simulink model "BusTest"  (R2022b)
settings: Solver=VariableStepAuto  StartTime=0.0  StopTime=10.0  RelTol=1e-3
undefined symbols (not defined in the file): AB_SAMPLE, ABC_SAMPLE, AC_SAMPLE, C_Fault_IaConfirmCnt_u16, C_Fault_IaInstantFaultCoeff_f32, C_Fault_IaInstantFaultDiagEn_u8, C_Fault_IaInstantFaultLevel_u8, ParamCfg_LaValueDefault_u16, ParamCfg_SampleMode_u16
libraries: simulink x4
settings Model: Creator=ZYH  LastModifiedBy=ZYH

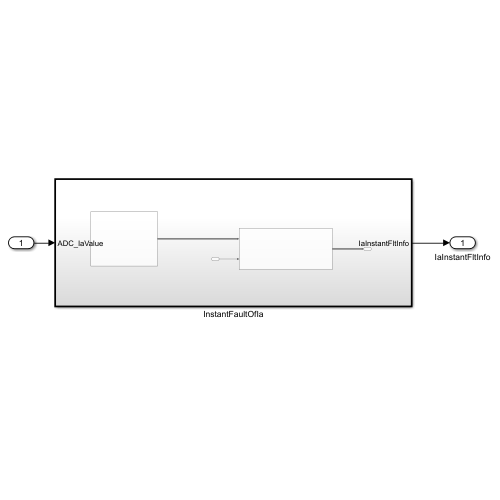
[thumbnail: Simulink's stored preview of the top-level diagram]
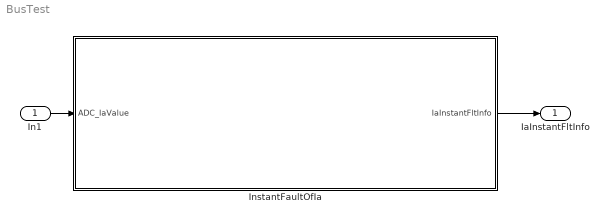
== system BusTest ==
  In1 : Inport
  InstantFaultOfIa : Subsystem  TreatAsAtomicUnit=on
      settings: RTWSystemCode=Nonreusable function
  IaInstantFltInfo : Outport
  wires:
  In1/1 -> InstantFaultOfIa/1(ADC_IaValue)
  InstantFaultOfIa/1(IaInstantFltInfo) -> IaInstantFltInfo/1

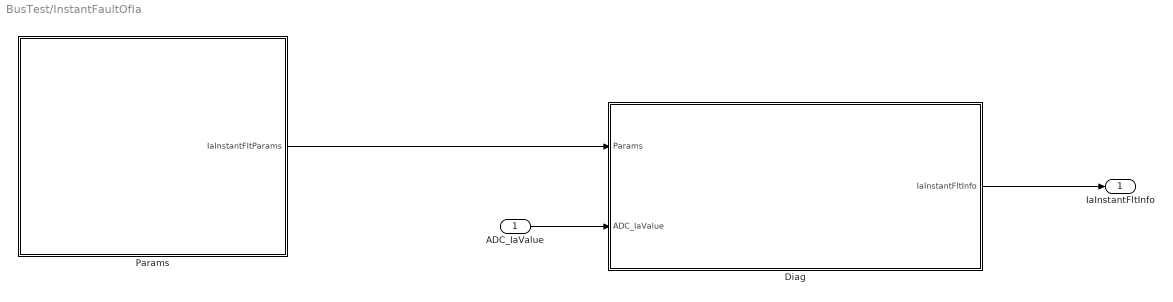
== system BusTest/InstantFaultOfIa ==
  ADC_IaValue : Inport
  Diag : Subsystem
  Params : Subsystem
  IaInstantFltInfo : Outport
  wires:
  Params/1(IaInstantFltParams) -> Diag/1(Params)
  ADC_IaValue/1 -> Diag/2(ADC_IaValue)
  Diag/1(IaInstantFltInfo) -> IaInstantFltInfo/1

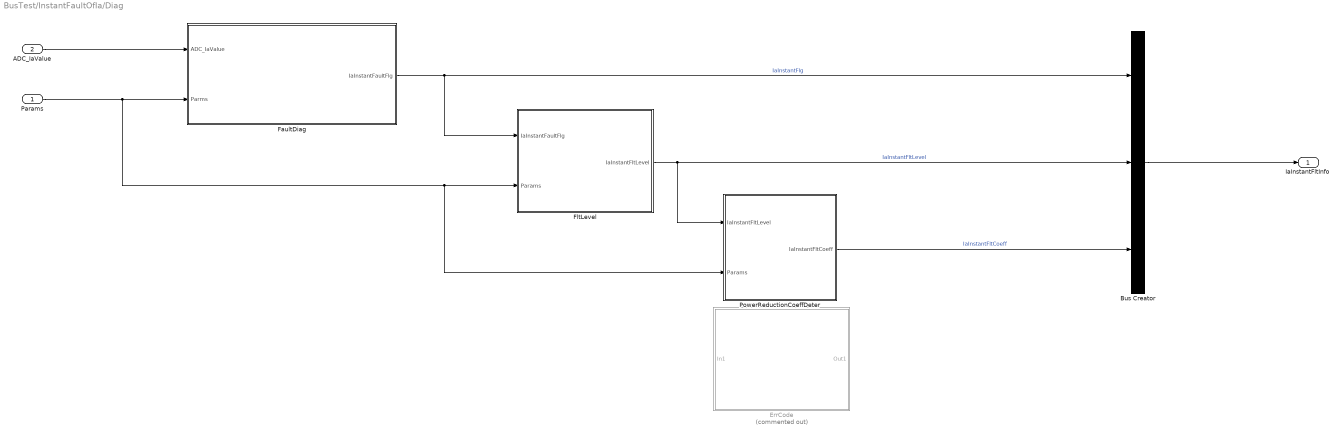
== system BusTest/InstantFaultOfIa/Diag ==
  Params : Inport
  ADC_IaValue : Inport  Port=2
  Bus Creator : BusCreator  Inputs=3  OutDataTypeStr=Bus: FaultBus
      settings: InheritFromInputs=off
  ErrCode : Subsystem  Commented=on
  FaultDiag : Subsystem
  FltLevel : Subsystem
  PowerReductionCoeffDeter : Subsystem
  IaInstantFltInfo : Outport
  wires:
  Params/1 -> PowerReductionCoeffDeter/2(Params), FltLevel/2(Params), FaultDiag/2(Parms)
  ADC_IaValue/1 -> FaultDiag/1(ADC_IaValue)
  FaultDiag/1(IaInstantFaultFlg) -> FltLevel/1(IaInstantFaultFlg), Bus Creator/1  "IaInstantFlg"
  PowerReductionCoeffDeter/1(IaInstantFltCoeff) -> Bus Creator/3  "IaInstantFltCoeff"
  FltLevel/1(IaInstantFltLevel) -> PowerReductionCoeffDeter/1(IaInstantFltLevel), Bus Creator/2  "IaInstantFltLevel"
  Bus Creator/1 -> IaInstantFltInfo/1

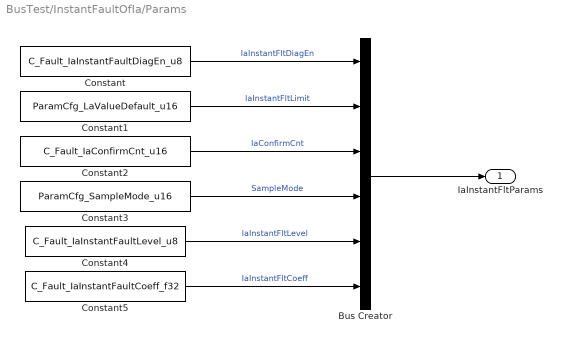
== system BusTest/InstantFaultOfIa/Params ==
  Bus Creator : BusCreator  Inputs=6
  Constant : Constant  Value=C_Fault_IaInstantFaultDiagEn_u8
  Constant1 : Constant  Value=ParamCfg_LaValueDefault_u16
  Constant2 : Constant  Value=C_Fault_IaConfirmCnt_u16  OutDataTypeStr=uint16
  Constant3 : Constant  Value=ParamCfg_SampleMode_u16
  Constant4 : Constant  Value=C_Fault_IaInstantFaultLevel_u8
  Constant5 : Constant  Value=C_Fault_IaInstantFaultCoeff_f32
  IaInstantFltParams : Outport
  wires:
  Constant1/1 -> Bus Creator/2  "IaInstantFltLimit"
  Constant/1 -> Bus Creator/1  "IaInstantFltDiagEn"
  Constant2/1 -> Bus Creator/3  "IaConfirmCnt"
  Bus Creator/1 -> IaInstantFltParams/1
  Constant3/1 -> Bus Creator/4  "SampleMode"
  Constant4/1 -> Bus Creator/5  "IaInstantFltLevel"
  Constant5/1 -> Bus Creator/6  "IaInstantFltCoeff"

== system BusTest/InstantFaultOfIa/Diag/ErrCode ==
  In1 : Inport
  Out1 : Outport
  wires:
  In1/1 -> Out1/1

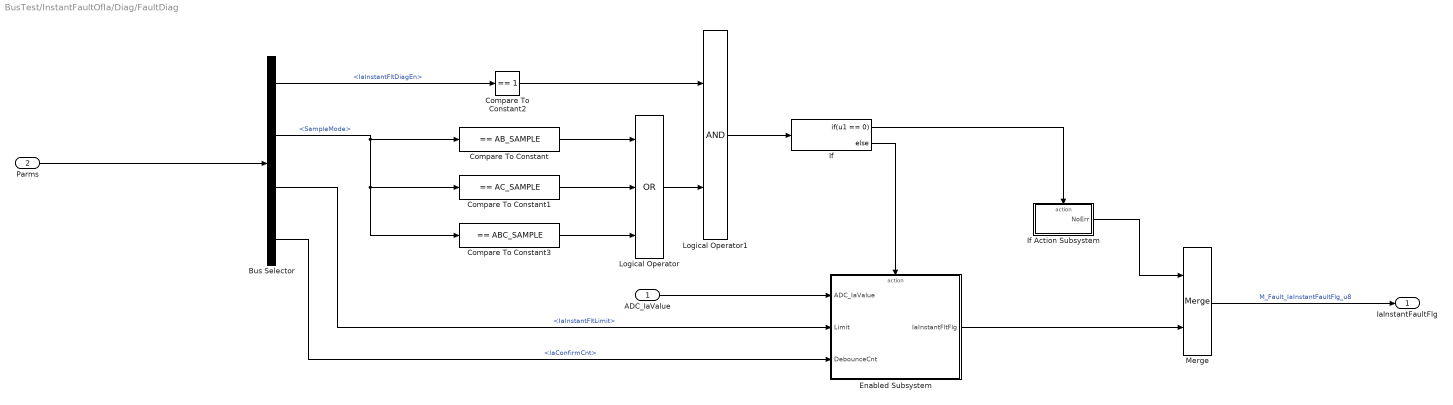
== system BusTest/InstantFaultOfIa/Diag/FaultDiag ==
  ADC_IaValue : Inport
  Parms : Inport  Port=2
  Bus Selector : BusSelector  OutputSignals=IaInstantFltDiagEn,SampleMode,IaInstantFltLimit,IaConfirmCnt
  Compare To Constant : simulink/Logic and Bit Operations/Compare To Constant  relop===  const=AB_SAMPLE  OutDataTypeStr=boolean
  Compare To Constant1 : simulink/Logic and Bit Operations/Compare To Constant  relop===  const=AC_SAMPLE  OutDataTypeStr=boolean
  Compare To Constant2 : simulink/Logic and Bit Operations/Compare To Constant  relop===  const=1  OutDataTypeStr=boolean
  Compare To Constant3 : simulink/Logic and Bit Operations/Compare To Constant  relop===  const=ABC_SAMPLE  OutDataTypeStr=boolean
  Enabled Subsystem : Subsystem  TreatAsAtomicUnit=on
  If : If  IfExpression=u1 == 0
  If Action Subsystem : Subsystem  TreatAsAtomicUnit=on
  Logical Operator : Logic  Operator=OR  Inputs=3  AllPortsSameDT=off  OutDataTypeStr=boolean
  Logical Operator1 : Logic  AllPortsSameDT=off  OutDataTypeStr=boolean
  Merge : Merge
  IaInstantFaultFlg : Outport
  wires:
  ADC_IaValue/1 -> Enabled Subsystem/1(ADC_IaValue)
  Bus Selector/4 -> Enabled Subsystem/3(DebounceCnt)  "<IaConfirmCnt>"
  Compare To Constant2/1 -> Logical Operator1/1
  Bus Selector/2 -> Compare To Constant3/1, Compare To Constant1/1, Compare To Constant/1  "<SampleMode>"
  Bus Selector/1 -> Compare To Constant2/1  "<IaInstantFltDiagEn>"
  Logical Operator/1 -> Logical Operator1/2
  Compare To Constant/1 -> Logical Operator/1
  Logical Operator1/1 -> If/1
  Compare To Constant3/1 -> Logical Operator/3
  Bus Selector/3 -> Enabled Subsystem/2(Limit)  "<IaInstantFltLimit>"
  Enabled Subsystem/1(IaInstantFltFlg) -> Merge/2
  If/2 -> Enabled Subsystem/Action
  Compare To Constant1/1 -> Logical Operator/2
  If Action Subsystem/1(NoErr) -> Merge/1
  If/1 -> If Action Subsystem/Action
  Parms/1 -> Bus Selector/1
  Merge/1 -> IaInstantFaultFlg/1  "M_Fault_IaInstantFaultFlg_u8"

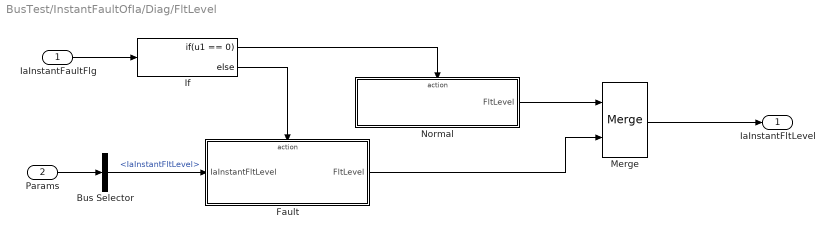
== system BusTest/InstantFaultOfIa/Diag/FltLevel ==
  IaInstantFaultFlg : Inport
  Params : Inport  Port=2
  Bus Selector : BusSelector  OutputSignals=IaInstantFltLevel
  Fault : Subsystem  TreatAsAtomicUnit=on
  If : If  IfExpression=u1 == 0
  Merge : Merge
  Normal : Subsystem  TreatAsAtomicUnit=on
  IaInstantFltLevel : Outport
  wires:
  IaInstantFaultFlg/1 -> If/1
  If/1 -> Normal/Action
  If/2 -> Fault/Action
  Params/1 -> Bus Selector/1
  Bus Selector/1 -> Fault/1(IaInstantFltLevel)  "<IaInstantFltLevel>"
  Normal/1(FltLevel) -> Merge/1
  Fault/1(FltLevel) -> Merge/2
  Merge/1 -> IaInstantFltLevel/1

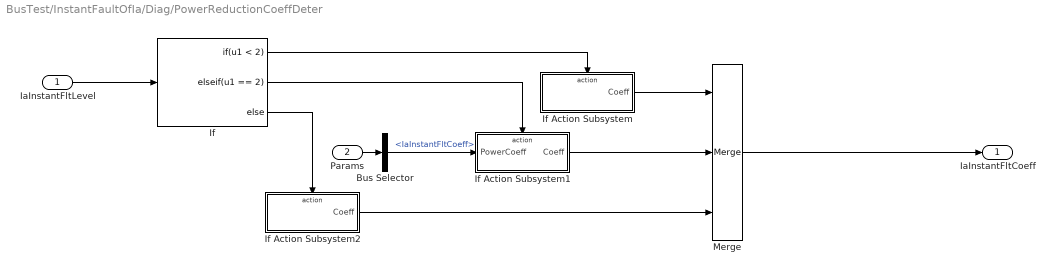
== system BusTest/InstantFaultOfIa/Diag/PowerReductionCoeffDeter ==
  IaInstantFltLevel : Inport
  Params : Inport  Port=2
  Bus Selector : BusSelector  OutputSignals=IaInstantFltCoeff
  If : If  IfExpression=u1 < 2  ElseIfExpressions=u1 == 2
  If Action Subsystem : Subsystem  TreatAsAtomicUnit=on
  If Action Subsystem1 : Subsystem  TreatAsAtomicUnit=on
  If Action Subsystem2 : Subsystem  TreatAsAtomicUnit=on
  Merge : Merge  Inputs=3
  IaInstantFltCoeff : Outport
  wires:
  IaInstantFltLevel/1 -> If/1
  If/1 -> If Action Subsystem/Action
  If/2 -> If Action Subsystem1/Action
  If/3 -> If Action Subsystem2/Action
  If Action Subsystem/1(Coeff) -> Merge/1
  If Action Subsystem1/1(Coeff) -> Merge/2
  If Action Subsystem2/1(Coeff) -> Merge/3
  Merge/1 -> IaInstantFltCoeff/1
  Bus Selector/1 -> If Action Subsystem1/1(PowerCoeff)  "<IaInstantFltCoeff>"
  Params/1 -> Bus Selector/1

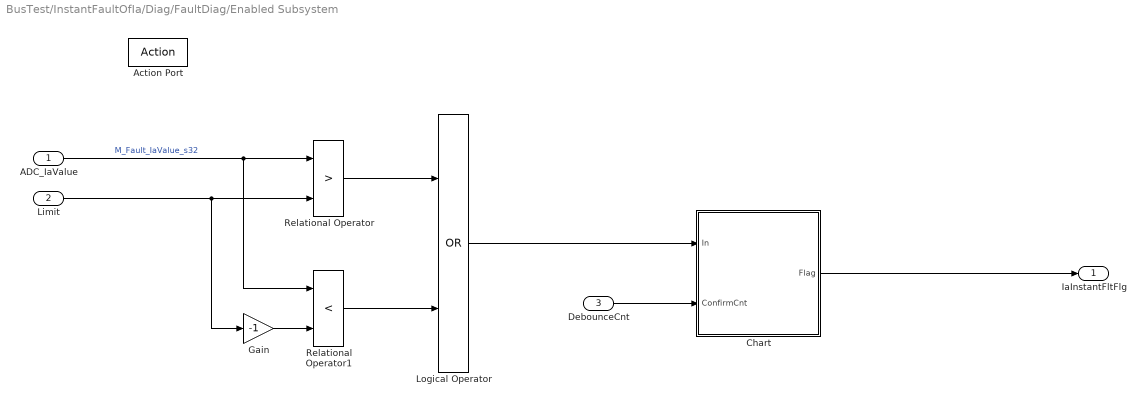
== system BusTest/InstantFaultOfIa/Diag/FaultDiag/Enabled Subsystem ==
  ADC_IaValue : Inport
  Limit : Inport  Port=2
  DebounceCnt : Inport  Port=3
  Action Port : ActionPort
  Chart : Stateflow chart  TreatAsAtomicUnit=on
      settings: RTWSystemCode=Inline
  Gain : Gain  Gain=-1  ParamDataTypeStr=single  OutDataTypeStr=single
  Logical Operator : Logic  Operator=OR  AllPortsSameDT=off  OutDataTypeStr=boolean
  Relational Operator : RelationalOperator  Operator=>  OutDataTypeStr=boolean  RndMeth=Simplest  InputSameDT=off
  Relational Operator1 : RelationalOperator  Operator=<  OutDataTypeStr=boolean  RndMeth=Simplest  InputSameDT=off
  IaInstantFltFlg : Outport
  wires:
  Logical Operator/1 -> Chart/1(In)
  Relational Operator/1 -> Logical Operator/1
  Gain/1 -> Relational Operator1/2
  ADC_IaValue/1 -> Relational Operator1/1, Relational Operator/1  "M_Fault_IaValue_s32"
  Relational Operator1/1 -> Logical Operator/2
  Limit/1 -> Gain/1, Relational Operator/2
  DebounceCnt/1 -> Chart/2(ConfirmCnt)
  Chart/1(Flag) -> IaInstantFltFlg/1

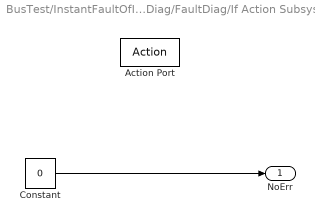
== system BusTest/InstantFaultOfIa/Diag/FaultDiag/If Action Subsystem ==
  Action Port : ActionPort
  Constant : Constant  Value=0  OutDataTypeStr=uint8
  NoErr : Outport
  wires:
  Constant/1 -> NoErr/1

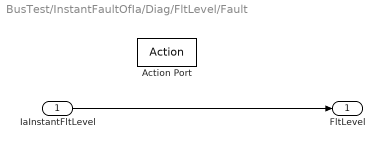
== system BusTest/InstantFaultOfIa/Diag/FltLevel/Fault ==
  IaInstantFltLevel : Inport
  Action Port : ActionPort
  FltLevel : Outport
  wires:
  IaInstantFltLevel/1 -> FltLevel/1

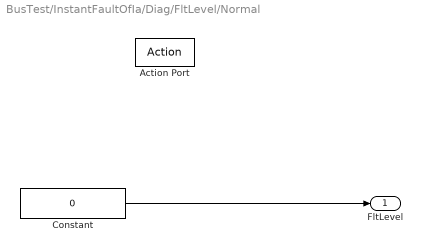
== system BusTest/InstantFaultOfIa/Diag/FltLevel/Normal ==
  Action Port : ActionPort
  Constant : Constant  Value=0  OutDataTypeStr=uint8
  FltLevel : Outport
  wires:
  Constant/1 -> FltLevel/1

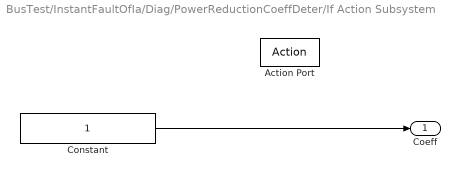
== system BusTest/InstantFaultOfIa/Diag/PowerReductionCoeffDeter/If Action Subsystem ==
  Action Port : ActionPort
  Constant : Constant  OutDataTypeStr=single
  Coeff : Outport
  wires:
  Constant/1 -> Coeff/1

== system BusTest/InstantFaultOfIa/Diag/PowerReductionCoeffDeter/If Action Subsystem1 ==
  PowerCoeff : Inport
  Action Port : ActionPort
  Coeff : Outport
  wires:
  PowerCoeff/1 -> Coeff/1

== system BusTest/InstantFaultOfIa/Diag/PowerReductionCoeffDeter/If Action Subsystem2 ==
  Action Port : ActionPort
  Constant : Constant  Value=0  OutDataTypeStr=single
  Coeff : Outport
  wires:
  Constant/1 -> Coeff/1

== stateflow chart BusTest/InstantFaultOfIa/Diag/FaultDiag/Enabled Subsystem/Chart ==
  (default) -> (junction 2)
  (junction 2) -> (junction 4) [order 1] : [In == true]
  (junction 2) -> (junction 18) [order 2] : {Flag = false;
      | Cnt = 0;}
  (junction 4) -> (junction 6) : {Cnt = Cnt+1}
  (junction 6) -> (junction 11) [order 1] : [Cnt > ConfirmCnt]
  (junction 6) -> (junction 15) [order 2]
  (junction 11) -> (junction 13) : {Flag = true;
      | Cnt = 0;}
  (junction 15) -> (junction 18)
  (junction 13) -> (junction 15)
  (junction 18) -> (junction 21)
  data: In input; Cnt local uint16 size=1 =0; ConfirmCnt input; Flag output uint8 =0
